simulink model "System_simulation_v1"  (R2025b)
settings: Solver=VariableStepAuto  StartTime=0.0  StopTime=150  RelTol=1e-3
undefined symbols (not defined in the file): Inertia, Inertia_inv, Kd_craft, Kp_craft, q_ref
libraries: aerolibutil x2, sharedutil x2, matrix_library x1
settings Model: Creator=erika  LastModifiedBy=erika

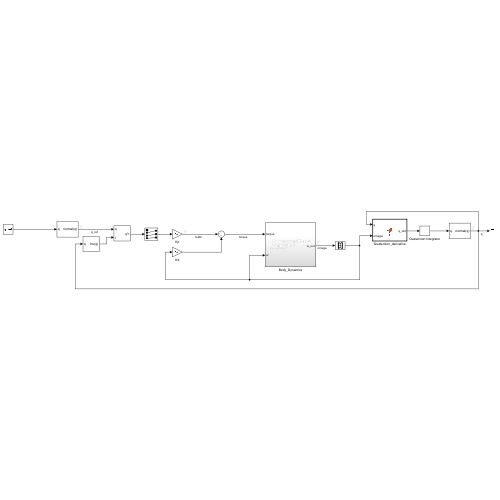
[thumbnail: Simulink's stored preview of the top-level diagram]
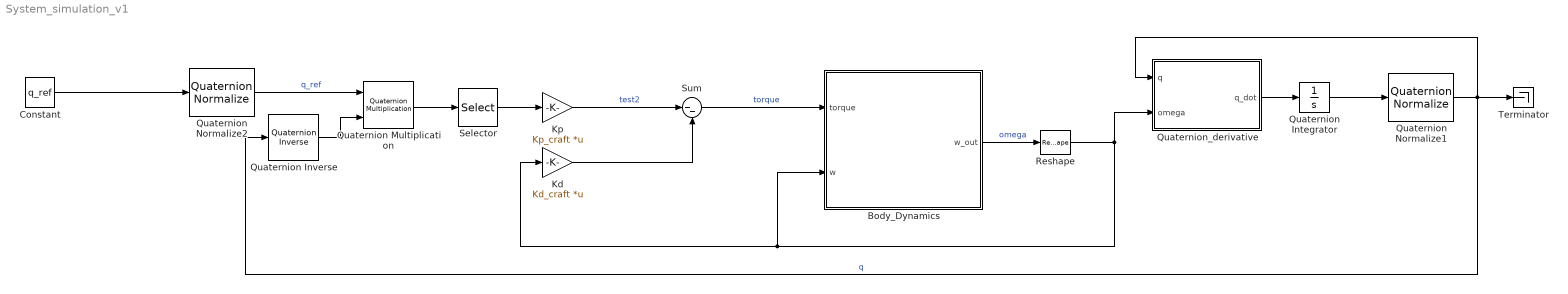
== system System_simulation_v1 ==
  Body_Dynamics : Subsystem
  Constant : Constant  Value=q_ref
  Kd : Gain  Gain=Kd_craft  Multiplication=Matrix(K*u)
  Kp : Gain  Gain=Kp_craft  Multiplication=Matrix(K*u)
  Quaternion Inverse : aerolibutil/Quaternion Inverse
  Quaternion Multiplication : aerolibutil/Quaternion Multiplication
  Quaternion Normalize1 : sharedutil/Quaternion Normalize  aMode=aMode
  Quaternion Normalize2 : sharedutil/Quaternion Normalize  aMode=aMode
  Quaternion Integrator : Integrator  InitialCondition=[1; 0; 0; 0]
  Quaternion_derivative : MATLAB Function  TreatAsAtomicUnit=on
  Reshape : Reshape  OutputDimensionality=Column vector (2-D)
  Selector : Selector  InputPortWidth=4  IndexOptions=Index vector (dialog)  Indices=[2 3 4]  OutputSizes=1
  Sum : Sum  Inputs=|--
  Terminator : Terminator
  wires:
  Quaternion Integrator/1 -> Quaternion Normalize1/1
  Quaternion_derivative/1(q_dot) -> Quaternion Integrator/1
  Kp/1 -> Sum/1  "test2"
  Kd/1 -> Sum/2
  Constant/1 -> Quaternion Normalize2/1
  Quaternion Multiplication/1 -> Selector/1
  Selector/1 -> Kp/1
  Sum/1 -> Body_Dynamics/1(torque)  "torque"
  Body_Dynamics/1(w_out) -> Reshape/1  "omega"
  Quaternion Normalize1/1 -> Quaternion_derivative/1(q), Quaternion Inverse/1, Terminator/1  "q"
  Reshape/1 -> Quaternion_derivative/2(omega), Kd/1, Body_Dynamics/2(w)
  Quaternion Normalize2/1 -> Quaternion Multiplication/1  "q_ref"
  Quaternion Inverse/1 -> Quaternion Multiplication/2

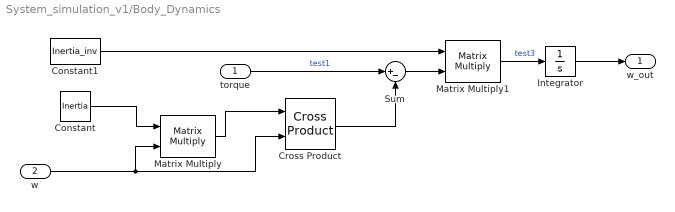
== system System_simulation_v1/Body_Dynamics ==
  torque : Inport
  w : Inport  Port=2
  Constant : Constant  Value=Inertia
  Constant1 : Constant  Value=Inertia_inv
  Cross Product : matrix_library/Cross Product
  Integrator : Integrator
  Matrix Multiply : Product  Multiplication=Matrix(*)
  Matrix Multiply1 : Product  Multiplication=Matrix(*)
  Sum : Sum  Inputs=|+-
  w_out : Outport  PortDimensions=[3 1]
  wires:
  w/1 -> Matrix Multiply/2, Cross Product/2
  Cross Product/1 -> Sum/2
  Constant/1 -> Matrix Multiply/1
  Matrix Multiply/1 -> Cross Product/1
  torque/1 -> Sum/1  "test1"
  Sum/1 -> Matrix Multiply1/2
  Matrix Multiply1/1 -> Integrator/1  "test3"
  Integrator/1 -> w_out/1
  Constant1/1 -> Matrix Multiply1/1

== matlab function System_simulation_v1/Quaternion_derivative ==
  data: q input size=[4 1]; q_dot output size=[4 1]; omega input size=[3 1]
function q_dot = f(q, omega)

    wx = omega(1);
    wy = omega(2);
    wz = omega(3);

    Omega = [ 0   -wx  -wy  -wz;
              wx   0    wz  -wy;
              wy  -wz   0    wx;
              wz   wy  -wx   0  ];

    q_dot = 0.5 * Omega * q;
end
